simulink model "state_traj"  (Simulink 7.1)
settings: Solver=ode23  StartTime=0.0  StopTime=t(1)  MaxStep=1e-2  RelTol=1e-6
values from neighbouring files (symbols this model uses):
  a_max = 1    [assignment1.m]    (also in assignment3.m = p0 = -; assignment4.m = p0 = -)
  g = 9.81    [MPCsimulink.m]    (also in assignment4.m; pend_init.m; setupOptimization.m)
  l = 0.345    [MPCsimulink.m]    (also in assignment4.m; loaddym.m = fgetl(fid); pend_init.m)
  p0 = -1.5    [assignment1.m]    (also in assignment5.m = -0.8)
undefined symbols (not defined in the file or in its folder): tSwitch
settings Model: Creator=pontusg  LastModifiedBy=pontusg  ExtModeAutoUpdateStatusClock=off
settings DebuggingCC: SaveWithParameterizedLinksMsg=none
settings GRTTargetCC: TargetFcnLib=ansi_tfl_tmw.mat

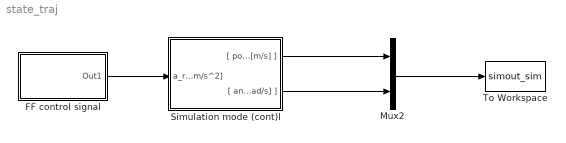
== system state_traj ==
  FF control signal : Subsystem
  Mux2 : Mux  Inputs=2
  Simulation mode (cont)l : Subsystem
  To Workspace : ToWorkspace  VariableName=simout_sim  SampleTime=-1  SaveFormat=Structure With Time
  wires:
  Mux2/1 -> To Workspace/1
  FF control signal/1(Out1) -> Simulation mode (cont)l/1(a_ref [m/s^2])
  Simulation mode (cont)l/1("[ pos [m] , vel [m/s] ]") -> Mux2/1
  Simulation mode (cont)l/2("[ ang [rad] , angVel [rad/s] ]") -> Mux2/2

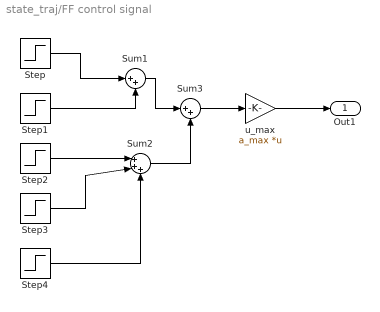
== system state_traj/FF control signal ==
  Step : Step  Time=0  SampleTime=0
  Step1 : Step  Time=tSwitch(1)  After=-2  SampleTime=0
  Step2 : Step  Time=tSwitch(2)  After=2  SampleTime=0
  Step3 : Step  Time=tSwitch(3)  After=-2  SampleTime=0
  Step4 : Step  Time=tSwitch(4)  SampleTime=0
  Sum1 : Sum  Inputs=|++  OutDataType=sfix(16)  OutScaling=2^0
  Sum2 : Sum  Inputs=|+++  OutDataType=sfix(16)  OutScaling=2^0
  Sum3 : Sum  Inputs=|++  OutDataType=sfix(16)  OutScaling=2^0
  u_max : Gain  Gain=a_max  Multiplication=Matrix(K*u) (u vector)  ParameterDataType=sfix(16)  ParameterScaling=2^0  OutDataType=sfix(16)  OutScaling=2^0
  Out1 : Outport  OutDataType=sfix(16)  OutScaling=2^0
  wires:
  Step/1 -> Sum1/1
  Step1/1 -> Sum1/2
  Step2/1 -> Sum2/1
  Sum1/1 -> Sum3/1
  Sum2/1 -> Sum3/2
  Step3/1 -> Sum2/2
  Step4/1 -> Sum2/3
  Sum3/1 -> u_max/1
  u_max/1 -> Out1/1

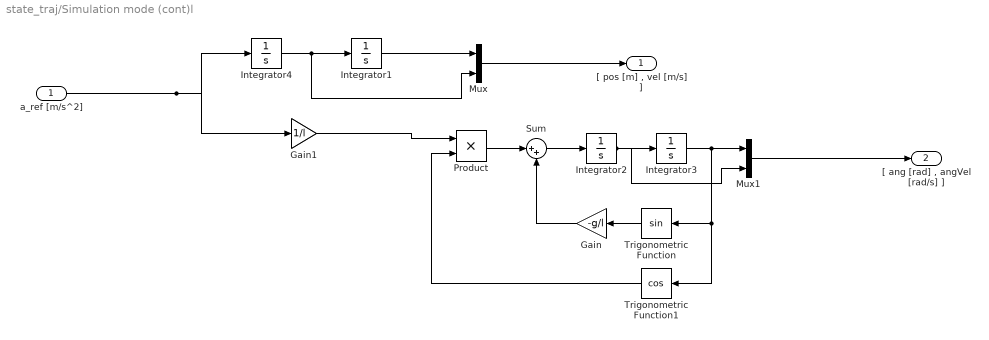
== system state_traj/Simulation mode (cont)l ==
  a_ref [m/s^2] : Inport  OutDataType=sfix(16)  OutScaling=2^0
  Gain : Gain  Orientation=left  Gain=-g/l  ParameterDataType=sfix(16)  ParameterScaling=2^0  OutDataType=sfix(16)  OutScaling=2^0
  Gain1 : Gain  Gain=1/l  ParameterDataType=sfix(16)  ParameterScaling=2^0  OutDataType=sfix(16)  OutScaling=2^0
  Integrator1 : Integrator  InitialCondition=p0
  Integrator2 : Integrator
  Integrator3 : Integrator
  Integrator4 : Integrator
  Mux : Mux  Inputs=2
  Mux1 : Mux  Inputs=2
  Product : Product  OutDataType=sfix(16)  OutScaling=2^0  RndMeth=Zero
  Sum : Sum  Inputs=|++  OutDataType=sfix(16)  OutScaling=2^0
  Trigonometric Function : Trigonometry  Orientation=left
  Trigonometric Function1 : Trigonometry  Orientation=left  Operator=cos
  "[ pos [m] , vel [m/s] ]" : Outport  OutDataType=sfix(16)  OutScaling=2^0
  "[ ang [rad] , angVel [rad/s] ]" : Outport  Port=2  OutDataType=sfix(16)  OutScaling=2^0
  wires:
  Gain/1 -> Sum/2
  Trigonometric Function/1 -> Gain/1
  Trigonometric Function1/1 -> Product/2
  Product/1 -> Sum/1
  Gain1/1 -> Product/1
  a_ref [m/s^2]/1 -> Integrator4/1, Gain1/1
  Mux1/1 -> "[ ang [rad] , angVel [rad/s] ]"/1
  Mux/1 -> "[ pos [m] , vel [m/s] ]"/1
  Sum/1 -> Integrator2/1
  Integrator3/1 -> Trigonometric Function1/1, Trigonometric Function/1, Mux1/1
  Integrator2/1 -> Mux1/2, Integrator3/1
  Integrator1/1 -> Mux/1
  Integrator4/1 -> Mux/2, Integrator1/1
